simulink model "Exp2_ControlSystemDemo"  (R2017b)
settings: Solver=ode4  StartTime=0.0  StopTime=2000  FixedStep=0.001  RelTol=1e-3
InitFcn:
  | Init_control;
values from neighbouring files (symbols this model uses):
  KiPitchAttitude = 0.0552303199591522 / kFactor    (= 0.0460252666326)    [Init_control.m]
  KiPitchRate = 0.460338699849681 / kFactor    (= 0.383615583208)    [Init_control.m]
  KiRollAttitude = 0.0552303199591522 / kFactor    (= 0.0460252666326)    [Init_control.m]
  KiRollRate = 0.460338699849681 / kFactor    (= 0.383615583208)    [Init_control.m]
  KiYawRate = 0.460338699849681 / kFactor    (= 0.383615583208)    [Init_control.m]
  KpPitchAttitude = 0.630138625117681 / kFactor    (= 0.525115520931)    [Init_control.m]
  KpPitchRate = 1.31533836563383 / kFactor    (= 1.09611530469)    [Init_control.m]
  KpRollAttitude = 0.630138625117681 / kFactor    (= 0.525115520931)    [Init_control.m]
  KpRollRate = 1.31533836563383 / kFactor    (= 1.09611530469)    [Init_control.m]
  KpYawRate = 1.31533836563383 / kFactor    (= 1.09611530469)    [Init_control.m]
undefined symbols (not defined in the file or in its folder): earthRadius, ModelInit_RPM, ModelParam_envAltitude, ModelParam_GlobalNoiseGainSwitch, ModelParam_GPSLatLong, ModelParam_motorCr, ModelParam_motorJm, ModelParam_motorMinThr, ModelParam_motorT, ModelParam_motorWb, ModelParam_rotorCm, ModelParam_rotorCt, ModelParam_uavCCm, ModelParam_uavCd, ModelParam_uavDearo, ModelParam_uavJ, ModelParam_uavMass, ModelParam_uavR, ModelParam_uavType, Receive, Send
libraries: simulink x6, aerolibfltsims x4, aerolib6dof2 x1, aerolibanimutils x1
(part 2 of 2)

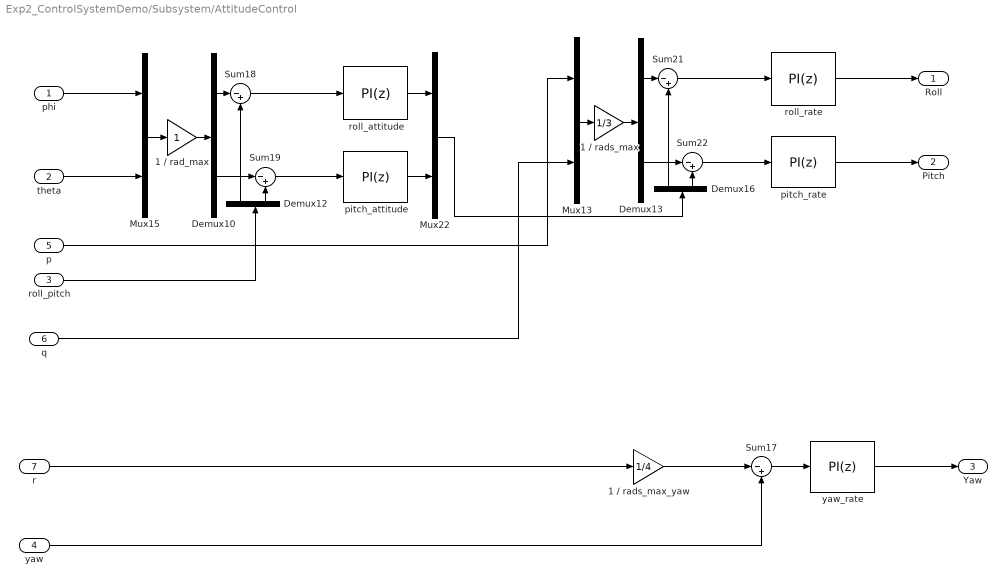
== system Exp2_ControlSystemDemo/Subsystem/AttitudeControl ==
  phi : Inport
  theta : Inport  Port=2
  roll_pitch : Inport  Port=3
  yaw : Inport  Port=4
  p : Inport  Port=5
  q : Inport  Port=6
  r : Inport  Port=7
  1 / rad_max : Gain
  1 / rads_max : Gain  Gain=1/3
  1 / rads_max_yaw : Gain  Gain=1/4
  Demux{10,12..13,16} (4 alike) : Demux  Outputs=2
  Mux13 : Mux  Inputs=2
  Mux15 : Mux  Inputs=2
  Mux22 : Mux  Inputs=2
  Sum{17..19,21..22} (5 alike) : Sum  Inputs=|-+
  pitch_attitude : simulink/Continuous/PID Controller  Controller=PI  TimeDomain=Discrete-time  SampleTime=-1  IntegratorMethod=Forward Euler  FilterMethod=Forward Euler  Form=Parallel  UseFilter=on  ControllerParametersSource=internal  P=KpPitchAttitude  I=KiPitchAttitude  D=0.01  N=100  InitialConditionSource=internal  InitialConditionForIntegrator=0  InitialConditionForFilter=0  ExternalReset=none  LimitOutput=on  UpperSaturationLimit=1  LowerSaturationLimit=-1  LinearizeAsGain=on  AntiWindupMode=back-calculation  Kb=1  TrackingMode=off  Kt=1  PParamMin=[]  PParamMax=[]  IParamMin=[]  IParamMax=[]  DParamMin=[]  DParamMax=[]  NParamMin=[]  NParamMax=[]  KbParamMin=[]  KbParamMax=[]  KtParamMin=[]  KtParamMax=[]  POutMin=[]  POutMax=[]  IOutMin=[]  IOutMax=[]  DOutMin=[]  DOutMax=[]  NOutMin=[]  NOutMax=[]  KbOutMin=[]  KbOutMax=[]  KtOutMin=[]  KtOutMax=[]  IntegratorOutMin=[]  IntegratorOutMax=[]  FilterOutMin=[]  FilterOutMax=[]  SumOutMin=[]  SumOutMax=[]  SumI1OutMin=[]  SumI1OutMax=[]  SumI2OutMin=[]  SumI2OutMax=[]  SumI3OutMin=[]  SumI3OutMax=[]  SumDOutMin=[]  SumDOutMax=[]  SaturationOutMin=[]  SaturationOutMax=[]  IntegratorContinuousStateAttributes=''  IntegratorStateMustResolveToSignalObject=off  IntegratorRTWStateStorageClass=Auto  FilterContinuousStateAttributes=''  FilterStateMustResolveToSignalObject=off  FilterRTWStateStorageClass=Auto  DifferentiatorICPrevScaledInput=0  DifferentiatorOutMin=[]  DifferentiatorOutMax=[]
  pitch_rate : simulink/Continuous/PID Controller  Controller=PI  TimeDomain=Discrete-time  SampleTime=-1  IntegratorMethod=Forward Euler  FilterMethod=Forward Euler  Form=Parallel  UseFilter=on  ControllerParametersSource=internal  P=KpPitchRate  I=KiPitchRate  D=0.0024  N=100  InitialConditionSource=internal  InitialConditionForIntegrator=0  InitialConditionForFilter=0  ExternalReset=none  LimitOutput=on  UpperSaturationLimit=1  LowerSaturationLimit=-1  LinearizeAsGain=on  AntiWindupMode=back-calculation  Kb=1  TrackingMode=off  Kt=1  PParamMin=[]  PParamMax=[]  IParamMin=[]  IParamMax=[]  DParamMin=[]  DParamMax=[]  NParamMin=[]  NParamMax=[]  KbParamMin=[]  KbParamMax=[]  KtParamMin=[]  KtParamMax=[]  POutMin=[]  POutMax=[]  IOutMin=[]  IOutMax=[]  DOutMin=[]  DOutMax=[]  NOutMin=[]  NOutMax=[]  KbOutMin=[]  KbOutMax=[]  KtOutMin=[]  KtOutMax=[]  IntegratorOutMin=[]  IntegratorOutMax=[]  FilterOutMin=[]  FilterOutMax=[]  SumOutMin=[]  SumOutMax=[]  SumI1OutMin=[]  SumI1OutMax=[]  SumI2OutMin=[]  SumI2OutMax=[]  SumI3OutMin=[]  SumI3OutMax=[]  SumDOutMin=[]  SumDOutMax=[]  SaturationOutMin=[]  SaturationOutMax=[]  IntegratorContinuousStateAttributes=''  IntegratorStateMustResolveToSignalObject=off  IntegratorRTWStateStorageClass=Auto  FilterContinuousStateAttributes=''  FilterStateMustResolveToSignalObject=off  FilterRTWStateStorageClass=Auto  DifferentiatorICPrevScaledInput=0  DifferentiatorOutMin=[]  DifferentiatorOutMax=[]
  roll_attitude : simulink/Continuous/PID Controller  Controller=PI  TimeDomain=Discrete-time  SampleTime=-1  IntegratorMethod=Forward Euler  FilterMethod=Forward Euler  Form=Parallel  UseFilter=on  ControllerParametersSource=internal  P=KpRollAttitude  I=KiRollAttitude  D=0.01  N=100  InitialConditionSource=internal  InitialConditionForIntegrator=0  InitialConditionForFilter=0  ExternalReset=none  LimitOutput=on  UpperSaturationLimit=1  LowerSaturationLimit=-1  LinearizeAsGain=on  AntiWindupMode=back-calculation  Kb=1  TrackingMode=off  Kt=1  PParamMin=[]  PParamMax=[]  IParamMin=[]  IParamMax=[]  DParamMin=[]  DParamMax=[]  NParamMin=[]  NParamMax=[]  KbParamMin=[]  KbParamMax=[]  KtParamMin=[]  KtParamMax=[]  POutMin=[]  POutMax=[]  IOutMin=[]  IOutMax=[]  DOutMin=[]  DOutMax=[]  NOutMin=[]  NOutMax=[]  KbOutMin=[]  KbOutMax=[]  KtOutMin=[]  KtOutMax=[]  IntegratorOutMin=[]  IntegratorOutMax=[]  FilterOutMin=[]  FilterOutMax=[]  SumOutMin=[]  SumOutMax=[]  SumI1OutMin=[]  SumI1OutMax=[]  SumI2OutMin=[]  SumI2OutMax=[]  SumI3OutMin=[]  SumI3OutMax=[]  SumDOutMin=[]  SumDOutMax=[]  SaturationOutMin=[]  SaturationOutMax=[]  IntegratorContinuousStateAttributes=''  IntegratorStateMustResolveToSignalObject=off  IntegratorRTWStateStorageClass=Auto  FilterContinuousStateAttributes=''  FilterStateMustResolveToSignalObject=off  FilterRTWStateStorageClass=Auto  DifferentiatorICPrevScaledInput=0  DifferentiatorOutMin=[]  DifferentiatorOutMax=[]
  roll_rate : simulink/Continuous/PID Controller  Controller=PI  TimeDomain=Discrete-time  SampleTime=-1  IntegratorMethod=Forward Euler  FilterMethod=Forward Euler  Form=Parallel  UseFilter=on  ControllerParametersSource=internal  P=KpRollRate  I=KiRollRate  D=0.0024  N=100  InitialConditionSource=internal  InitialConditionForIntegrator=0  InitialConditionForFilter=0  ExternalReset=none  LimitOutput=on  UpperSaturationLimit=1  LowerSaturationLimit=-1  LinearizeAsGain=on  AntiWindupMode=back-calculation  Kb=1  TrackingMode=off  Kt=1  PParamMin=[]  PParamMax=[]  IParamMin=[]  IParamMax=[]  DParamMin=[]  DParamMax=[]  NParamMin=[]  NParamMax=[]  KbParamMin=[]  KbParamMax=[]  KtParamMin=[]  KtParamMax=[]  POutMin=[]  POutMax=[]  IOutMin=[]  IOutMax=[]  DOutMin=[]  DOutMax=[]  NOutMin=[]  NOutMax=[]  KbOutMin=[]  KbOutMax=[]  KtOutMin=[]  KtOutMax=[]  IntegratorOutMin=[]  IntegratorOutMax=[]  FilterOutMin=[]  FilterOutMax=[]  SumOutMin=[]  SumOutMax=[]  SumI1OutMin=[]  SumI1OutMax=[]  SumI2OutMin=[]  SumI2OutMax=[]  SumI3OutMin=[]  SumI3OutMax=[]  SumDOutMin=[]  SumDOutMax=[]  SaturationOutMin=[]  SaturationOutMax=[]  IntegratorContinuousStateAttributes=''  IntegratorStateMustResolveToSignalObject=off  IntegratorRTWStateStorageClass=Auto  FilterContinuousStateAttributes=''  FilterStateMustResolveToSignalObject=off  FilterRTWStateStorageClass=Auto  DifferentiatorICPrevScaledInput=0  DifferentiatorOutMin=[]  DifferentiatorOutMax=[]
  yaw_rate : simulink/Continuous/PID Controller  Controller=PI  TimeDomain=Discrete-time  SampleTime=-1  IntegratorMethod=Forward Euler  FilterMethod=Forward Euler  Form=Parallel  UseFilter=on  ControllerParametersSource=internal  P=KpYawRate  I=KiYawRate  D=0  N=100  InitialConditionSource=internal  InitialConditionForIntegrator=0  InitialConditionForFilter=0  ExternalReset=none  LimitOutput=on  UpperSaturationLimit=1  LowerSaturationLimit=-1  LinearizeAsGain=on  AntiWindupMode=back-calculation  Kb=1  TrackingMode=off  Kt=1  PParamMin=[]  PParamMax=[]  IParamMin=[]  IParamMax=[]  DParamMin=[]  DParamMax=[]  NParamMin=[]  NParamMax=[]  KbParamMin=[]  KbParamMax=[]  KtParamMin=[]  KtParamMax=[]  POutMin=[]  POutMax=[]  IOutMin=[]  IOutMax=[]  DOutMin=[]  DOutMax=[]  NOutMin=[]  NOutMax=[]  KbOutMin=[]  KbOutMax=[]  KtOutMin=[]  KtOutMax=[]  IntegratorOutMin=[]  IntegratorOutMax=[]  FilterOutMin=[]  FilterOutMax=[]  SumOutMin=[]  SumOutMax=[]  SumI1OutMin=[]  SumI1OutMax=[]  SumI2OutMin=[]  SumI2OutMax=[]  SumI3OutMin=[]  SumI3OutMax=[]  SumDOutMin=[]  SumDOutMax=[]  SaturationOutMin=[]  SaturationOutMax=[]  IntegratorContinuousStateAttributes=''  IntegratorStateMustResolveToSignalObject=off  IntegratorRTWStateStorageClass=Auto  FilterContinuousStateAttributes=''  FilterStateMustResolveToSignalObject=off  FilterRTWStateStorageClass=Auto  DifferentiatorICPrevScaledInput=0  DifferentiatorOutMin=[]  DifferentiatorOutMax=[]
  Roll : Outport
  Pitch : Outport  Port=2
  Yaw : Outport  Port=3
  wires:
  r/1 -> 1 / rads_max_yaw/1
  q/1 -> Mux13/2
  Mux22/1 -> Demux16/1
  yaw_rate/1 -> Yaw/1
  phi/1 -> Mux15/1
  Mux15/1 -> 1 / rad_max/1
  theta/1 -> Mux15/2
  1 / rads_max_yaw/1 -> Sum17/1
  roll_rate/1 -> Roll/1
  Sum19/1 -> pitch_attitude/1
  pitch_attitude/1 -> Mux22/2
  roll_attitude/1 -> Mux22/1
  Demux16/1 -> Sum21/2
  yaw/1 -> Sum17/2
  roll_pitch/1 -> Demux12/1
  Demux16/2 -> Sum22/2
  Demux12/1 -> Sum18/2
  Demux12/2 -> Sum19/2
  p/1 -> Mux13/1
  Demux10/1 -> Sum18/1
  Demux10/2 -> Sum19/1
  1 / rad_max/1 -> Demux10/1
  Sum18/1 -> roll_attitude/1
  pitch_rate/1 -> Pitch/1
  Mux13/1 -> 1 / rads_max/1
  Sum22/1 -> pitch_rate/1
  Sum17/1 -> yaw_rate/1
  Demux13/1 -> Sum21/1
  Demux13/2 -> Sum22/1
  1 / rads_max/1 -> Demux13/1
  Sum21/1 -> roll_rate/1

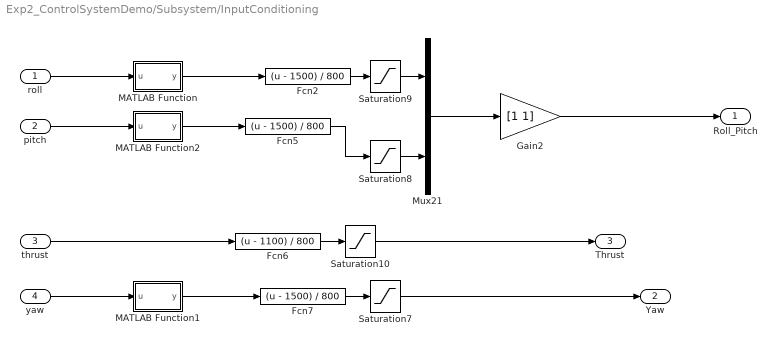
== system Exp2_ControlSystemDemo/Subsystem/InputConditioning ==
  roll : Inport
  pitch : Inport  Port=2
  thrust : Inport  Port=3
  yaw : Inport  Port=4
  Fcn2 : Fcn  Expr=(u - 1500) / 800
  Fcn5 : Fcn  Expr=(u - 1500) / 800
  Fcn6 : Fcn  Expr=(u - 1100) / 800
  Fcn7 : Fcn  Expr=(u - 1500) / 800
  Gain2 : Gain  Gain=[1 1]  OutDataTypeStr=Inherit: Inherit via back propagation
  MATLAB Function : MATLAB Function  TreatAsAtomicUnit=on
  MATLAB Function1 : MATLAB Function  TreatAsAtomicUnit=on
  MATLAB Function2 : MATLAB Function  TreatAsAtomicUnit=on
  Mux21 : Mux  Inputs=2
  Saturation10 : Saturate  UpperLimit=1  LowerLimit=0
  Saturation7 : Saturate  UpperLimit=1  LowerLimit=-1
  Saturation8 : Saturate  UpperLimit=1  LowerLimit=-1
  Saturation9 : Saturate  UpperLimit=1  LowerLimit=-1
  Roll_Pitch : Outport
  Yaw : Outport  Port=2
  Thrust : Outport  Port=3
  wires:
  Saturation10/1 -> Thrust/1
  Saturation7/1 -> Yaw/1
  Gain2/1 -> Roll_Pitch/1
  Mux21/1 -> Gain2/1
  Saturation8/1 -> Mux21/2
  Fcn6/1 -> Saturation10/1
  Fcn2/1 -> Saturation9/1
  Fcn5/1 -> Saturation8/1
  Saturation9/1 -> Mux21/1
  Fcn7/1 -> Saturation7/1
  pitch/1 -> MATLAB Function2/1(u)
  MATLAB Function1/1(y) -> Fcn7/1
  thrust/1 -> Fcn6/1
  roll/1 -> MATLAB Function/1(u)
  MATLAB Function2/1(y) -> Fcn5/1
  MATLAB Function/1(y) -> Fcn2/1
  yaw/1 -> MATLAB Function1/1(u)

== system Exp2_ControlSystemDemo/Quadcopter Dynamics/Battery Model/__InputSSForSFun__ ==
  PWMin : Inport
  __UniqueOutportName__1__ : Outport
  wires:
  PWMin/1 -> __UniqueOutportName__1__/1

== system Exp2_ControlSystemDemo/Quadcopter Dynamics/Battery Model/__OutputSSForSFun__ ==
  __UniqueInportName__1__ : Inport
  __UniqueInportName__2__ : Inport  Port=2
  __UniqueInportName__3__ : Inport  Port=3
  Mux1 : BusCreator  Inputs=3
  Battery Model Bus : Outport
  wires:
  __UniqueInportName__1__/1 -> Mux1/1  "PWMOut"
  __UniqueInportName__2__/1 -> Mux1/2  "cellVol"
  __UniqueInportName__3__/1 -> Mux1/3  "remCapa"
  Mux1/1 -> Battery Model Bus/1

== system Exp2_ControlSystemDemo/Quadcopter Dynamics/Environment Model/__InputSSForSFun__ ==
  6DOF Bus : Inport
  temporaryBusSelectName_1 : BusSelector  OutputSignals=Ve,Xe,Eular(rad),DCM,Vb,wb,dwb/dt
  __UniqueOutportName__1__ : Outport
  __UniqueOutportName__2__ : Outport  Port=2
  __UniqueOutportName__3__ : Outport  Port=3
  __UniqueOutportName__4__ : Outport  Port=4
  __UniqueOutportName__5__ : Outport  Port=5
  __UniqueOutportName__6__ : Outport  Port=6
  __UniqueOutportName__7__ : Outport  Port=7
  wires:
  6DOF Bus/1 -> temporaryBusSelectName_1/1
  temporaryBusSelectName_1/1 -> __UniqueOutportName__1__/1  "<Ve>"
  temporaryBusSelectName_1/2 -> __UniqueOutportName__2__/1  "<Xe>"
  temporaryBusSelectName_1/3 -> __UniqueOutportName__3__/1  "<Eular(rad)>"
  temporaryBusSelectName_1/4 -> __UniqueOutportName__4__/1  "<DCM>"
  temporaryBusSelectName_1/5 -> __UniqueOutportName__5__/1  "<Vb>"
  temporaryBusSelectName_1/6 -> __UniqueOutportName__6__/1  "<wb>"
  temporaryBusSelectName_1/7 -> __UniqueOutportName__7__/1  "<dwb/dt>"

== system Exp2_ControlSystemDemo/Quadcopter Dynamics/Environment Model/__OutputSSForSFun__ ==
  __UniqueInportName__1__ : Inport
  __UniqueInportName__2__ : Inport  Port=2
  __UniqueInportName__3__ : Inport  Port=3
  __UniqueInportName__4__ : Inport  Port=4
  __UniqueInportName__5__ : Inport  Port=5
  __UniqueInportName__6__ : Inport  Port=6
  __UniqueInportName__7__ : Inport  Port=7
  Mux1 : BusCreator  Inputs=7
  Environment Model Bus : Outport
  wires:
  __UniqueInportName__1__/1 -> Mux1/1  "PosGPS"
  __UniqueInportName__2__/1 -> Mux1/2  "gravity"
  __UniqueInportName__3__/1 -> Mux1/3  "TempC"
  __UniqueInportName__4__/1 -> Mux1/4  "AirPressure"
  __UniqueInportName__5__/1 -> Mux1/5  "Rho"
  __UniqueInportName__6__/1 -> Mux1/6  "Windb"
  __UniqueInportName__7__/1 -> Mux1/7  "Wind"
  Mux1/1 -> Environment Model Bus/1

== system Exp2_ControlSystemDemo/Quadcopter Dynamics/Fail Model/__InputSSForSFun__ ==
  6DOF Bus : Inport
  temporaryBusSelectName_1 : BusSelector  OutputSignals=Ve,Xe,Eular(rad),DCM,Vb,wb,dwb/dt
  __UniqueOutportName__1__ : Outport
  __UniqueOutportName__2__ : Outport  Port=2
  __UniqueOutportName__3__ : Outport  Port=3
  __UniqueOutportName__4__ : Outport  Port=4
  __UniqueOutportName__5__ : Outport  Port=5
  __UniqueOutportName__6__ : Outport  Port=6
  __UniqueOutportName__7__ : Outport  Port=7
  wires:
  6DOF Bus/1 -> temporaryBusSelectName_1/1
  temporaryBusSelectName_1/1 -> __UniqueOutportName__1__/1  "<Ve>"
  temporaryBusSelectName_1/2 -> __UniqueOutportName__2__/1  "<Xe>"
  temporaryBusSelectName_1/3 -> __UniqueOutportName__3__/1  "<Eular(rad)>"
  temporaryBusSelectName_1/4 -> __UniqueOutportName__4__/1  "<DCM>"
  temporaryBusSelectName_1/5 -> __UniqueOutportName__5__/1  "<Vb>"
  temporaryBusSelectName_1/6 -> __UniqueOutportName__6__/1  "<wb>"
  temporaryBusSelectName_1/7 -> __UniqueOutportName__7__/1  "<dwb/dt>"

== system Exp2_ControlSystemDemo/Quadcopter Dynamics/Fail Model/__OutputSSForSFun__ ==
  __UniqueInportName__1__ : Inport
  __UniqueInportName__2__ : Inport  Port=2
  __UniqueInportName__3__ : Inport  Port=3
  Mux1 : BusCreator  Inputs=3
  Fail Model Bus : Outport
  wires:
  __UniqueInportName__1__/1 -> Mux1/1  "m"
  __UniqueInportName__2__/1 -> Mux1/2  "J"
  __UniqueInportName__3__/1 -> Mux1/3  "dM"
  Mux1/1 -> Fail Model Bus/1

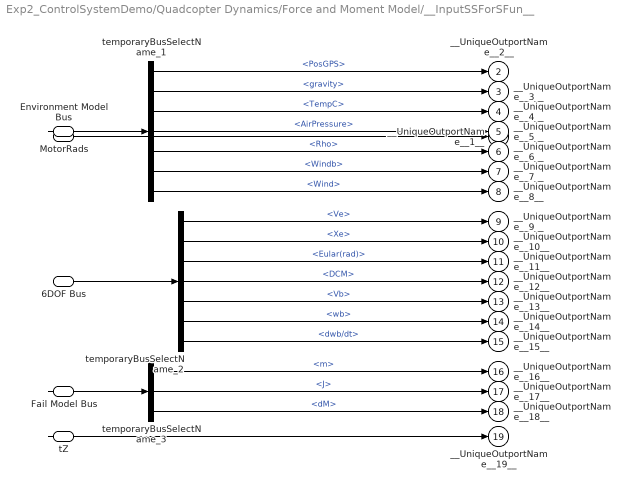
== system Exp2_ControlSystemDemo/Quadcopter Dynamics/Force and Moment Model/__InputSSForSFun__ ==
  MotorRads : Inport
  Environment Model Bus : Inport  Port=2
  6DOF Bus : Inport  Port=3
  Fail Model Bus : Inport  Port=4
  "tZ " : Inport  Port=5
  temporaryBusSelectName_1 : BusSelector  OutputSignals=PosGPS,gravity,TempC,AirPressure,Rho,Windb,Wind
  temporaryBusSelectName_2 : BusSelector  OutputSignals=Ve,Xe,Eular(rad),DCM,Vb,wb,dwb/dt
  temporaryBusSelectName_3 : BusSelector  OutputSignals=m,J,dM
  __UniqueOutportName__1__ : Outport
  __UniqueOutportName__2__ : Outport  Port=2
  __UniqueOutportName__3__ : Outport  Port=3
  __UniqueOutportName__4__ : Outport  Port=4
  __UniqueOutportName__5__ : Outport  Port=5
  __UniqueOutportName__6__ : Outport  Port=6
  __UniqueOutportName__7__ : Outport  Port=7
  __UniqueOutportName__8__ : Outport  Port=8
  __UniqueOutportName__9__ : Outport  Port=9
  __UniqueOutportName__10__ : Outport  Port=10
  __UniqueOutportName__11__ : Outport  Port=11
  __UniqueOutportName__12__ : Outport  Port=12
  __UniqueOutportName__13__ : Outport  Port=13
  __UniqueOutportName__14__ : Outport  Port=14
  __UniqueOutportName__15__ : Outport  Port=15
  __UniqueOutportName__16__ : Outport  Port=16
  __UniqueOutportName__17__ : Outport  Port=17
  __UniqueOutportName__18__ : Outport  Port=18
  __UniqueOutportName__19__ : Outport  Port=19
  wires:
  Environment Model Bus/1 -> temporaryBusSelectName_1/1
  6DOF Bus/1 -> temporaryBusSelectName_2/1
  Fail Model Bus/1 -> temporaryBusSelectName_3/1
  MotorRads/1 -> __UniqueOutportName__1__/1
  temporaryBusSelectName_1/1 -> __UniqueOutportName__2__/1  "<PosGPS>"
  temporaryBusSelectName_1/2 -> __UniqueOutportName__3__/1  "<gravity>"
  temporaryBusSelectName_1/3 -> __UniqueOutportName__4__/1  "<TempC>"
  temporaryBusSelectName_1/4 -> __UniqueOutportName__5__/1  "<AirPressure>"
  temporaryBusSelectName_1/5 -> __UniqueOutportName__6__/1  "<Rho>"
  temporaryBusSelectName_1/6 -> __UniqueOutportName__7__/1  "<Windb>"
  temporaryBusSelectName_1/7 -> __UniqueOutportName__8__/1  "<Wind>"
  temporaryBusSelectName_2/1 -> __UniqueOutportName__9__/1  "<Ve>"
  temporaryBusSelectName_2/2 -> __UniqueOutportName__10__/1  "<Xe>"
  temporaryBusSelectName_2/3 -> __UniqueOutportName__11__/1  "<Eular(rad)>"
  temporaryBusSelectName_2/4 -> __UniqueOutportName__12__/1  "<DCM>"
  temporaryBusSelectName_2/5 -> __UniqueOutportName__13__/1  "<Vb>"
  temporaryBusSelectName_2/6 -> __UniqueOutportName__14__/1  "<wb>"
  temporaryBusSelectName_2/7 -> __UniqueOutportName__15__/1  "<dwb/dt>"
  temporaryBusSelectName_3/1 -> __UniqueOutportName__16__/1  "<m>"
  temporaryBusSelectName_3/2 -> __UniqueOutportName__17__/1  "<J>"
  temporaryBusSelectName_3/3 -> __UniqueOutportName__18__/1  "<dM>"
  "tZ "/1 -> __UniqueOutportName__19__/1

== system Exp2_ControlSystemDemo/Quadcopter Dynamics/Force and Moment Model/__OutputSSForSFun__ ==
  __UniqueInportName__1__ : Inport
  __UniqueInportName__2__ : Inport  Port=2
  __UniqueInportName__3__ : Inport  Port=3
  Mux1 : BusCreator  Inputs=3
  Force and Moment Model Bus : Outport
  wires:
  __UniqueInportName__1__/1 -> Mux1/1  "Fb"
  __UniqueInportName__2__/1 -> Mux1/2  "Mb"
  __UniqueInportName__3__/1 -> Mux1/3  "landed"
  Mux1/1 -> Force and Moment Model Bus/1

== system Exp2_ControlSystemDemo/Quadcopter Dynamics/Motor Model/__InputSSForSFun__ ==
  Battery Model Bus : Inport
  temporaryBusSelectName_1 : BusSelector  OutputSignals=PWMOut,cellVol,remCapa
  __UniqueOutportName__1__ : Outport
  __UniqueOutportName__2__ : Outport  Port=2
  __UniqueOutportName__3__ : Outport  Port=3
  wires:
  Battery Model Bus/1 -> temporaryBusSelectName_1/1
  temporaryBusSelectName_1/1 -> __UniqueOutportName__1__/1  "<PWMOut>"
  temporaryBusSelectName_1/2 -> __UniqueOutportName__2__/1  "<cellVol>"
  temporaryBusSelectName_1/3 -> __UniqueOutportName__3__/1  "<remCapa>"

== system Exp2_ControlSystemDemo/Quadcopter Dynamics/Motor Model/__OutputSSForSFun__ ==
  __UniqueInportName__1__ : Inport
  MotorRads : Outport
  wires:
  __UniqueInportName__1__/1 -> MotorRads/1  "y"

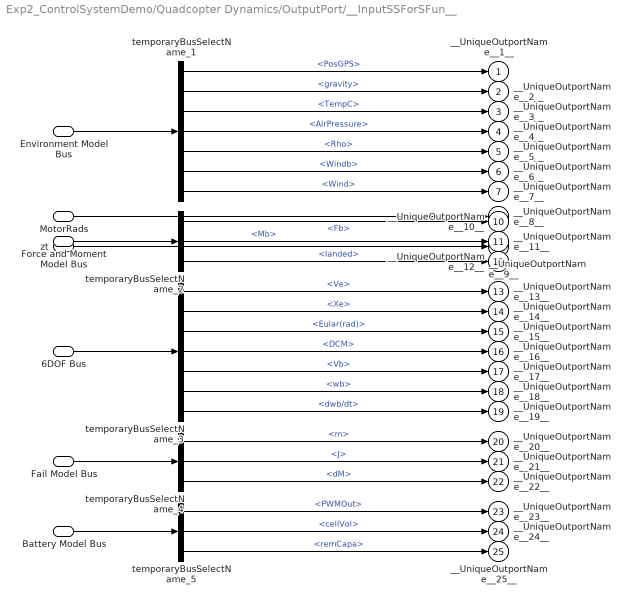
== system Exp2_ControlSystemDemo/Quadcopter Dynamics/OutputPort/__InputSSForSFun__ ==
  Environment Model Bus : Inport
  MotorRads : Inport  Port=2
  zt : Inport  Port=3
  Force and Moment Model Bus : Inport  Port=4
  6DOF Bus : Inport  Port=5
  Fail Model Bus : Inport  Port=6
  Battery Model Bus : Inport  Port=7
  temporaryBusSelectName_1 : BusSelector  OutputSignals=PosGPS,gravity,TempC,AirPressure,Rho,Windb,Wind
  temporaryBusSelectName_2 : BusSelector  OutputSignals=Fb,Mb,landed
  temporaryBusSelectName_3 : BusSelector  OutputSignals=Ve,Xe,Eular(rad),DCM,Vb,wb,dwb/dt
  temporaryBusSelectName_4 : BusSelector  OutputSignals=m,J,dM
  temporaryBusSelectName_5 : BusSelector  OutputSignals=PWMOut,cellVol,remCapa
  __UniqueOutportName__1__ : Outport
  __UniqueOutportName__2__ : Outport  Port=2
  __UniqueOutportName__3__ : Outport  Port=3
  __UniqueOutportName__4__ : Outport  Port=4
  __UniqueOutportName__5__ : Outport  Port=5
  __UniqueOutportName__6__ : Outport  Port=6
  __UniqueOutportName__7__ : Outport  Port=7
  __UniqueOutportName__8__ : Outport  Port=8
  __UniqueOutportName__9__ : Outport  Port=9
  __UniqueOutportName__10__ : Outport  Port=10
  __UniqueOutportName__11__ : Outport  Port=11
  __UniqueOutportName__12__ : Outport  Port=12
  __UniqueOutportName__13__ : Outport  Port=13
  __UniqueOutportName__14__ : Outport  Port=14
  __UniqueOutportName__15__ : Outport  Port=15
  __UniqueOutportName__16__ : Outport  Port=16
  __UniqueOutportName__17__ : Outport  Port=17
  __UniqueOutportName__18__ : Outport  Port=18
  __UniqueOutportName__19__ : Outport  Port=19
  __UniqueOutportName__20__ : Outport  Port=20
  __UniqueOutportName__21__ : Outport  Port=21
  __UniqueOutportName__22__ : Outport  Port=22
  __UniqueOutportName__23__ : Outport  Port=23
  __UniqueOutportName__24__ : Outport  Port=24
  __UniqueOutportName__25__ : Outport  Port=25
  wires:
  Environment Model Bus/1 -> temporaryBusSelectName_1/1
  Force and Moment Model Bus/1 -> temporaryBusSelectName_2/1
  6DOF Bus/1 -> temporaryBusSelectName_3/1
  Fail Model Bus/1 -> temporaryBusSelectName_4/1
  Battery Model Bus/1 -> temporaryBusSelectName_5/1
  temporaryBusSelectName_1/1 -> __UniqueOutportName__1__/1  "<PosGPS>"
  temporaryBusSelectName_1/2 -> __UniqueOutportName__2__/1  "<gravity>"
  temporaryBusSelectName_1/3 -> __UniqueOutportName__3__/1  "<TempC>"
  temporaryBusSelectName_1/4 -> __UniqueOutportName__4__/1  "<AirPressure>"
  temporaryBusSelectName_1/5 -> __UniqueOutportName__5__/1  "<Rho>"
  temporaryBusSelectName_1/6 -> __UniqueOutportName__6__/1  "<Windb>"
  temporaryBusSelectName_1/7 -> __UniqueOutportName__7__/1  "<Wind>"
  MotorRads/1 -> __UniqueOutportName__8__/1
  zt/1 -> __UniqueOutportName__9__/1
  temporaryBusSelectName_2/1 -> __UniqueOutportName__10__/1  "<Fb>"
  temporaryBusSelectName_2/2 -> __UniqueOutportName__11__/1  "<Mb>"
  temporaryBusSelectName_2/3 -> __UniqueOutportName__12__/1  "<landed>"
  temporaryBusSelectName_3/1 -> __UniqueOutportName__13__/1  "<Ve>"
  temporaryBusSelectName_3/2 -> __UniqueOutportName__14__/1  "<Xe>"
  temporaryBusSelectName_3/3 -> __UniqueOutportName__15__/1  "<Eular(rad)>"
  temporaryBusSelectName_3/4 -> __UniqueOutportName__16__/1  "<DCM>"
  temporaryBusSelectName_3/5 -> __UniqueOutportName__17__/1  "<Vb>"
  temporaryBusSelectName_3/6 -> __UniqueOutportName__18__/1  "<wb>"
  temporaryBusSelectName_3/7 -> __UniqueOutportName__19__/1  "<dwb/dt>"
  temporaryBusSelectName_4/1 -> __UniqueOutportName__20__/1  "<m>"
  temporaryBusSelectName_4/2 -> __UniqueOutportName__21__/1  "<J>"
  temporaryBusSelectName_4/3 -> __UniqueOutportName__22__/1  "<dM>"
  temporaryBusSelectName_5/1 -> __UniqueOutportName__23__/1  "<PWMOut>"
  temporaryBusSelectName_5/2 -> __UniqueOutportName__24__/1  "<cellVol>"
  temporaryBusSelectName_5/3 -> __UniqueOutportName__25__/1  "<remCapa>"

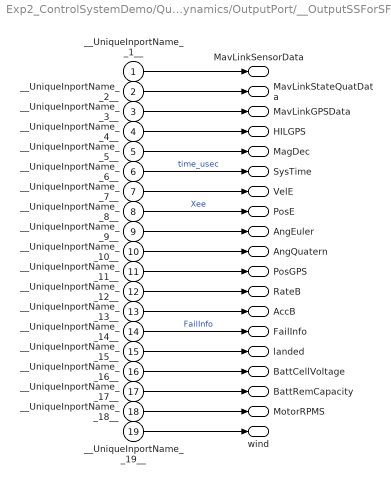
== system Exp2_ControlSystemDemo/Quadcopter Dynamics/OutputPort/__OutputSSForSFun__ ==
  __UniqueInportName__1__ : Inport
  __UniqueInportName__2__ : Inport  Port=2
  __UniqueInportName__3__ : Inport  Port=3
  __UniqueInportName__4__ : Inport  Port=4
  __UniqueInportName__5__ : Inport  Port=5
  __UniqueInportName__6__ : Inport  Port=6
  __UniqueInportName__7__ : Inport  Port=7
  __UniqueInportName__8__ : Inport  Port=8
  __UniqueInportName__9__ : Inport  Port=9
  __UniqueInportName__10__ : Inport  Port=10
  __UniqueInportName__11__ : Inport  Port=11
  __UniqueInportName__12__ : Inport  Port=12
  __UniqueInportName__13__ : Inport  Port=13
  __UniqueInportName__14__ : Inport  Port=14
  __UniqueInportName__15__ : Inport  Port=15
  __UniqueInportName__16__ : Inport  Port=16
  __UniqueInportName__17__ : Inport  Port=17
  __UniqueInportName__18__ : Inport  Port=18
  __UniqueInportName__19__ : Inport  Port=19
  MavLinkSensorData : Outport  OutDataTypeStr=Bus: MavLinkSensor  SampleTime=[-1 0]  BusOutputAsStruct=on
  MavLinkStateQuatData : Outport  Port=2  OutDataTypeStr=Bus: MavLinkStateQuat  SampleTime=[-1 0]  BusOutputAsStruct=on
  MavLinkGPSData : Outport  Port=3  OutDataTypeStr=Bus: MavLinkGPS  SampleTime=[-1 0]  BusOutputAsStruct=on
  HILGPS : Outport  Port=4  OutDataTypeStr=Bus: HILGPS  SampleTime=[-1 0]  BusOutputAsStruct=on
  MagDec : Outport  Port=5
  SysTime : Outport  Port=6
  VelE : Outport  Port=7
  PosE : Outport  Port=8
  AngEuler : Outport  Port=9
  AngQuatern : Outport  Port=10
  PosGPS : Outport  Port=11
  RateB : Outport  Port=12
  AccB : Outport  Port=13
  FailInfo : Outport  Port=14
  landed : Outport  Port=15
  BattCellVoltage : Outport  Port=16
  BattRemCapacity : Outport  Port=17
  MotorRPMS : Outport  Port=18
  wind : Outport  Port=19
  wires:
  __UniqueInportName__1__/1 -> MavLinkSensorData/1
  __UniqueInportName__2__/1 -> MavLinkStateQuatData/1
  __UniqueInportName__3__/1 -> MavLinkGPSData/1
  __UniqueInportName__4__/1 -> HILGPS/1
  __UniqueInportName__5__/1 -> MagDec/1
  __UniqueInportName__6__/1 -> SysTime/1  "time_usec"
  __UniqueInportName__7__/1 -> VelE/1
  __UniqueInportName__8__/1 -> PosE/1  "Xee"
  __UniqueInportName__9__/1 -> AngEuler/1
  __UniqueInportName__10__/1 -> AngQuatern/1
  __UniqueInportName__11__/1 -> PosGPS/1
  __UniqueInportName__12__/1 -> RateB/1
  __UniqueInportName__13__/1 -> AccB/1
  __UniqueInportName__14__/1 -> FailInfo/1  "FailInfo"
  __UniqueInportName__15__/1 -> landed/1
  __UniqueInportName__16__/1 -> BattCellVoltage/1
  __UniqueInportName__17__/1 -> BattRemCapacity/1
  __UniqueInportName__18__/1 -> MotorRPMS/1
  __UniqueInportName__19__/1 -> wind/1

== matlab function Exp2_ControlSystemDemo/Subsystem/InputConditioning/MATLAB Function ==
  data: u input; y output
function y = fcn(u)

 if(u>1600)
    y=u;
 else
     if(u<1400)
     y=u;
     else
         y=1500;
     end
 end

== matlab function Exp2_ControlSystemDemo/Subsystem/InputConditioning/MATLAB Function1 ==
  data: u input; y output
function y = fcn(u)

 if(u>1600)
    y=u;
 else
     if(u<1400)
     y=u;
     else
         y=1500;
     end
 end

== matlab function Exp2_ControlSystemDemo/Subsystem/InputConditioning/MATLAB Function2 ==
  data: u input; y output
function y = fcn(u)

 if(u>1600)
    y=u;
 else
     if(u<1400)
     y=u;
     else
         y=1500;
     end
 end

== matlab function Exp2_ControlSystemDemo/Subsystem/pwm_out1 ==
  data: Roll input; M1 output; Pitch input; Yaw input; Thrust input; M2 output; M3 output; M4 output
function [M1, M2, M3, M4] = motor_mixer(Roll, Pitch, Yaw, Thrust)

idle_PWM = 1000;

% Quad XROLL （根据QP里面的叉字形结构的文字）
% M1 = ((Pitch+ Yaw)+Thrust-Roll) * 1000 + idle_PWM;
 %M2 = ((Pitch - Yaw)+Thrust+Roll) * 1000 + idle_PWM;
 %M3 = ((Roll +Yaw) + Thrust-Pitch) * 1000 + idle_PWM;
 %M4 = ((-Roll - Pitch-Yaw) + Thrust) * 1000 + idle_PWM;
% M5 = 1000;
% M6 = 1000;
% M7 = 1000;
% M8 = 1000;
%qp上实际的输出
M1 = (Thrust+Pitch-Roll+Yaw) * 1000 + idle_PWM;
 M2 = (Thrust-Pitch +Roll+Yaw) * 1000 + idle_PWM;
 M3 = ( Thrust+Roll+Pitch-Yaw) * 1000 + idle_PWM;
 M4 = (Thrust-Roll- Pitch -Yaw) * 1000 + idle_PWM;
% Quad +
 %M1 = ((Pitch - Yaw) * Thrust / 2 + Thrust) * 1000 + idle_PWM;
 %M2 = ((-Roll + Yaw) * Thrust / 2 + Thrust) * 1000 + idle_PWM;
% M3 = ((-Pitch - Yaw) * Thrust / 2 + Thrust) * 1000 + idle_PWM;
 %M4 = ((Roll + Yaw) * Thrust / 2 + Thrust) * 1000 + idle_PWM;
% M5 = 1000;
% M6 = 1000;
% M7 = 1000;
% M8 = 1000;

% Hex X
% M1 = ((Pitch + Roll / 2 - Yaw) * Thrust / 2 + Thrust) * 1000 + idle_PWM;
% M2 = ((Pitch - Roll / 2 + Yaw) * Thrust / 2 + Thrust) * 1000 + idle_PWM;
% M3 = ((-Roll - Yaw) * Thrust / 2 + Thrust) * 1000 + idle_PWM;
% M4 = ((-Pitch - Roll / 2 + Yaw) * Thrust / 2 + Thrust) * 1000 + idle_PWM;
% M5 = ((-Pitch + Roll / 2 - Yaw) * Thrust / 2 + Thrust) * 1000 + idle_PWM;
% M6 = ((Roll + Yaw) * Thrust / 2 + Thrust) * 1000 + idle_PWM;
% M7 = 1000;
% M8 = 1000;

% Hex X (From Adam)
%M1 = uint16(single(((-Roll - Yaw) * Thrust / 3 + Thrust) * single(1000))) + idle_PWM;
%M2 = uint16(single(((Roll + Yaw) * Thrust / 3 + Thrust) * single(1000))) + idle_PWM;
%M3 = uint16(single(((Pitch + (Roll / 2) - Yaw) * Thrust / 3 + Thrust) * single(1000))) + idle_PWM;
%M4 = uint16(single(((-Pitch - (Roll / 2) + Yaw) * Thrust / 3 + Thrust) * single(1000))) + idle_PWM;
%M5 = uint16(single(((Pitch - (Roll / 2) + Yaw) * Thrust / 3 + Thrust) * single(1000))) + idle_PWM;
%M6 = uint16(single(((-Pitch + (Roll / 2) - Yaw) * Thrust / 3 + Thrust) * single(1000))) + idle_PWM;

% Hex X (Version 2)
% Roll/Yaw
% M1 = ((-Roll - Yaw) * Thrust / 2 + Thrust) * 1000 + idle_PWM;
% M2 = ((Roll + Yaw) * Thrust / 2 + Thrust) * 1000 + idle_PWM;
% % + Pitch/Roll
% M6 = ((Pitch + Roll / 2 - Yaw) * Thrust / 2 + Thrust) * 1000 + idle_PWM;
% M4 = ((Pitch - Roll / 2 + Yaw) * Thrust / 2 + Thrust) * 1000 + idle_PWM;
% % - Pitch/Roll
% M5 = ((-Pitch - Roll / 2 + Yaw) * Thrust / 2 + Thrust) * 1000 + idle_PWM;
% M3 = ((-Pitch + Roll / 2 - Yaw) * Thrust / 2 + Thrust) * 1000 + idle_PWM;
